simulink model "Quat_Test_v3"  (Simulink 7.5)
settings: Solver=FixedStepDiscrete  StartTime=0.0  StopTime=t(end)  FixedStep=SampleT  RelTol=1e-3
values from neighbouring files (symbols this model uses):
  apSampleTime = 0.01    [demoz2SlugsV5.m]
  QUAT_0 = DCM2Quat( R0 )    [demoz2SlugsV5.m]
  SampleT = 0.02    [demoz2SlugsV5.m]
undefined symbols (not defined in the file or in its folder): DiscIntNeverNeededParam
libraries: simulink x11, dspmtrx3 x1
settings Model: Creator=Robert  LastModifiedBy=Robert
settings DataIOCC: LimitDataPoints=off

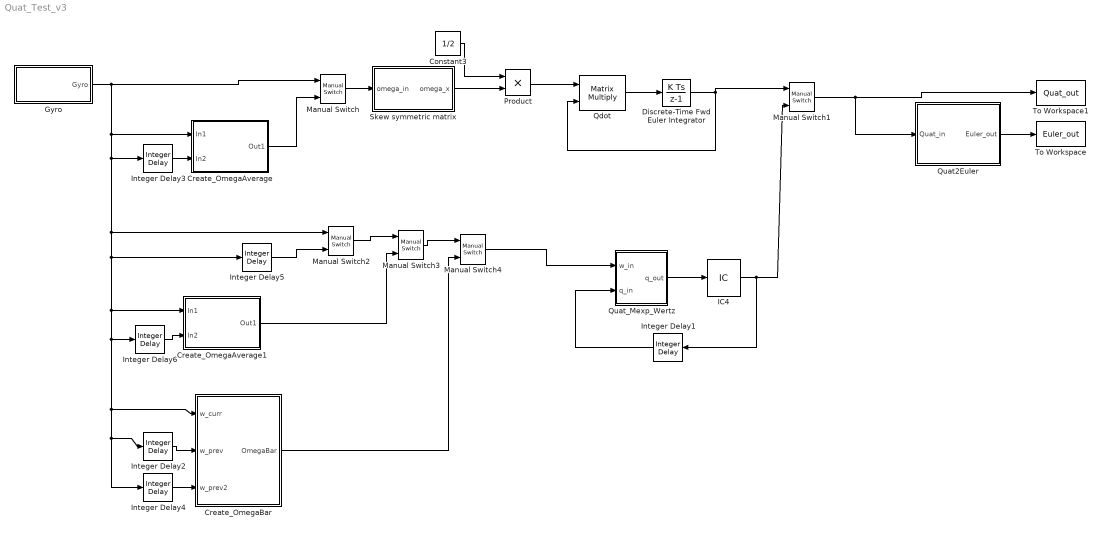
== system Quat_Test_v3 ==
  Constant3 : Constant  Value=1/2  OutDataTypeMode=single  OutDataType=fixdt(1, 16)  OutScaling=2^0  OutDataTypeStr=single
  Create_OmegaAverage : Subsystem
  Create_OmegaAverage1 : Subsystem
  Create_OmegaBar : Subsystem
  Discrete-Time Fwd Euler Integrator : DiscreteIntegrator  InitialCondition=QUAT_0  SampleTime=SampleT  OutDataTypeMode=single  OutDataType=fixdt(1, 16)  OutScaling=2^0  OutDataTypeStr=single  ICPrevOutput=DiscIntNeverNeededParam  ICPrevScaledInput=DiscIntNeverNeededParam
  Gyro : Subsystem
  IC4 : InitialCondition  Value=QUAT_0  SampleTime=apSampleTime
  Integer Delay{1..3,5..6} (5 alike) : simulink/Discrete/Integer Delay  vinit=0.0  samptime=-1  NumDelays=1
  Integer Delay4 : simulink/Discrete/Integer Delay  vinit=0.0  samptime=-1  NumDelays=2
  Manual Switch{,1,3..4} (4 alike) : simulink/Signal Routing/Manual Switch  SystemSampleTime=-1  sw=0  action=0  varsize=off
  Manual Switch2 : simulink/Signal Routing/Manual Switch  SystemSampleTime=-1  sw=1  action=0  varsize=off
  Product : Product  OutDataType=fixdt(1, 16)  OutScaling=2^0  RndMeth=Zero
  Qdot : Product  Multiplication=Matrix(*)  OutDataTypeMode=single  OutDataType=sfix(16)  OutScaling=2^0  OutDataTypeStr=single  SampleTime=SampleT
  Quat2Euler : Subsystem
  Quat_Mexp_Wertz : Subsystem
  Skew symmetric matrix : Subsystem
  To Workspace : ToWorkspace  VariableName=Euler_out  SampleTime=SampleT  SaveFormat=Structure
  To Workspace1 : ToWorkspace  VariableName=Quat_out  SampleTime=SampleT  SaveFormat=Structure
  wires:
  Discrete-Time Fwd Euler Integrator/1 -> Qdot/2, Manual Switch1/1
  Quat2Euler/1(Euler_out) -> To Workspace/1
  Qdot/1 -> Discrete-Time Fwd Euler Integrator/1
  Skew symmetric matrix/1(omega_x) -> Product/2
  Constant3/1 -> Product/1
  Product/1 -> Qdot/1
  Manual Switch/1 -> Skew symmetric matrix/1(omega_in)
  Gyro/1(Gyro) -> Manual Switch/1, Create_OmegaAverage/1(In1), Integer Delay3/1, Manual Switch2/1, Integer Delay5/1, Create_OmegaAverage1/1(In1), Integer Delay6/1, Create_OmegaBar/1(w_curr), Integer Delay2/1, Integer Delay4/1
  Integer Delay3/1 -> Create_OmegaAverage/2(In2)
  Create_OmegaAverage/1(Out1) -> Manual Switch/2
  Integer Delay5/1 -> Manual Switch2/2
  Manual Switch2/1 -> Manual Switch3/1
  Manual Switch3/1 -> Manual Switch4/1
  Integer Delay6/1 -> Create_OmegaAverage1/2(In2)
  Quat_Mexp_Wertz/1(q_out) -> IC4/1
  Manual Switch1/1 -> To Workspace1/1, Quat2Euler/1(Quat_in)
  IC4/1 -> Manual Switch1/2, Integer Delay1/1
  Integer Delay1/1 -> Quat_Mexp_Wertz/2(q_in)
  Manual Switch4/1 -> Quat_Mexp_Wertz/1(w_in)
  Create_OmegaAverage1/1(Out1) -> Manual Switch3/2
  Create_OmegaBar/1(OmegaBar) -> Manual Switch4/2
  Integer Delay2/1 -> Create_OmegaBar/2(w_prev)
  Integer Delay4/1 -> Create_OmegaBar/3(w_prev2)

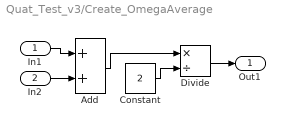
== system Quat_Test_v3/Create_OmegaAverage ==
  In1 : Inport
  In2 : Inport  Port=2
  Add : Sum  OutDataType=fixdt(1, 16)  OutScaling=2^-10
  Constant : Constant  Value=2  OutDataTypeMode=single  OutDataType=fixdt(1, 16)  OutScaling=2^0  OutDataTypeStr=single
  Divide : Product  Inputs=*/  OutDataType=fixdt(1, 16)  OutScaling=2^-10
  Out1 : Outport
  wires:
  Constant/1 -> Divide/2
  Add/1 -> Divide/1
  In1/1 -> Add/1
  In2/1 -> Add/2
  Divide/1 -> Out1/1

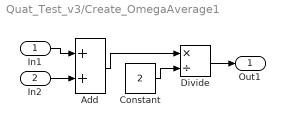
== system Quat_Test_v3/Create_OmegaAverage1 ==
  In1 : Inport
  In2 : Inport  Port=2
  Add : Sum  OutDataType=fixdt(1, 16)  OutScaling=2^-10
  Constant : Constant  Value=2  OutDataTypeMode=single  OutDataType=fixdt(1, 16)  OutScaling=2^0  OutDataTypeStr=single
  Divide : Product  Inputs=*/  OutDataType=fixdt(1, 16)  OutScaling=2^-10
  Out1 : Outport
  wires:
  Divide/1 -> Out1/1
  In2/1 -> Add/2
  In1/1 -> Add/1
  Add/1 -> Divide/1
  Constant/1 -> Divide/2

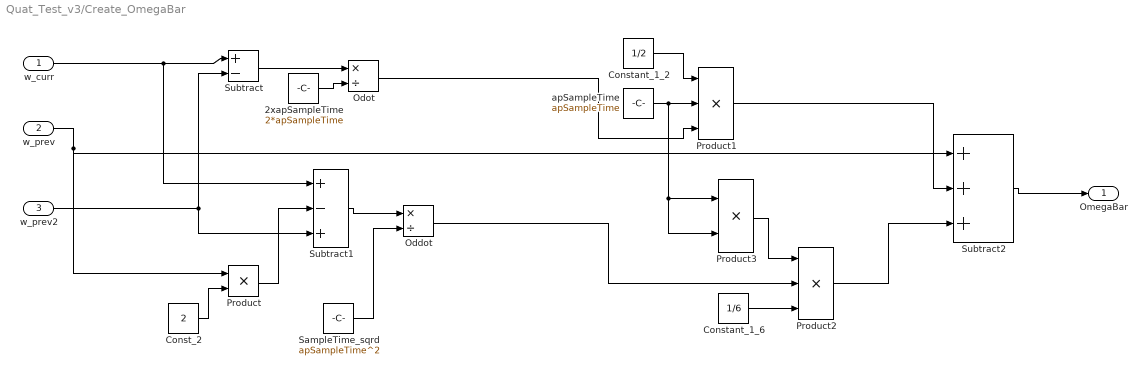
== system Quat_Test_v3/Create_OmegaBar ==
  w_curr : Inport
  w_prev : Inport  Port=2
  w_prev2 : Inport  Port=3
  2xapSampleTime : Constant  Value=2*apSampleTime  OutDataTypeMode=single  OutDataType=fixdt(1, 16)  OutScaling=2^0  OutDataTypeStr=single
  Const_2 : Constant  Value=2  OutDataTypeMode=single  OutDataType=fixdt(1, 16)  OutScaling=2^0  OutDataTypeStr=single
  Constant_1_2 : Constant  Value=1/2  OutDataTypeMode=single  OutDataType=fixdt(1, 16)  OutScaling=2^0  OutDataTypeStr=single
  Constant_1_6 : Constant  Value=1/6  OutDataTypeMode=single  OutDataType=fixdt(1, 16)  OutScaling=2^0  OutDataTypeStr=single
  Oddot : Product  Inputs=*/  OutDataType=fixdt(1, 16)  OutScaling=2^-10
  Odot : Product  Inputs=*/  OutDataType=fixdt(1, 16)  OutScaling=2^-10
  Product : Product  OutDataType=fixdt(1, 16)  OutScaling=2^0  RndMeth=Zero
  Product1 : Product  Inputs=3  OutDataType=fixdt(1, 16)  OutScaling=2^0  RndMeth=Zero
  Product2 : Product  Inputs=3  OutDataType=fixdt(1, 16)  OutScaling=2^0  RndMeth=Zero
  Product3 : Product  OutDataTypeMode=single  OutDataType=fixdt(1, 16)  OutScaling=2^0  OutDataTypeStr=single  SampleTime=apSampleTime  RndMeth=Zero
  SampleTime_sqrd : Constant  Value=apSampleTime^2  OutDataTypeMode=single  OutDataType=fixdt(1, 16)  OutScaling=2^0  OutDataTypeStr=single
  Subtract : Sum  Inputs=+-  OutDataType=fixdt(1, 16)  OutScaling=2^-10
  Subtract1 : Sum  Inputs=+-+  OutDataType=fixdt(1, 16)  OutScaling=2^-10
  Subtract2 : Sum  Inputs=+++  OutDataTypeMode=single  OutDataType=fixdt(1, 16)  OutScaling=2^-10  OutDataTypeStr=single
  apSampleTime : Constant  Value=apSampleTime  OutDataTypeMode=single  OutDataType=fixdt(1, 16)  OutScaling=2^0  OutDataTypeStr=single
  OmegaBar : Outport
  wires:
  w_prev/1 -> Product/1, Subtract2/1
  w_curr/1 -> Subtract/1, Subtract1/1
  w_prev2/1 -> Subtract/2, Subtract1/3
  Subtract/1 -> Odot/1
  2xapSampleTime/1 -> Odot/2
  SampleTime_sqrd/1 -> Oddot/2
  Subtract1/1 -> Oddot/1
  Const_2/1 -> Product/2
  Product/1 -> Subtract1/2
  Subtract2/1 -> OmegaBar/1
  Constant_1_2/1 -> Product1/1
  apSampleTime/1 -> Product1/2, Product3/1, Product3/2
  Odot/1 -> Product1/3
  Product1/1 -> Subtract2/2
  Constant_1_6/1 -> Product2/3
  Product3/1 -> Product2/1
  Oddot/1 -> Product2/2
  Product2/1 -> Subtract2/3

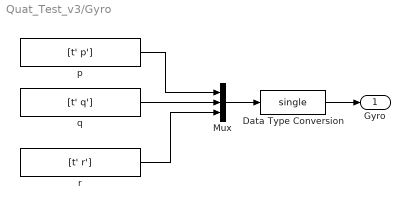
== system Quat_Test_v3/Gyro ==
  Data Type Conversion : DataTypeConversion  OutDataTypeMode=single  OutDataType=sfix(16)  OutScaling=2^0  OutDataTypeStr=single  SampleTime=SampleT
  Mux : Mux  Inputs=3
  p : FromWorkspace  VariableName=[t' p']  SampleTime=SampleT  Interpolate=off  OutputAfterFinalValue=Setting to zero
  q : FromWorkspace  VariableName=[t' q']  SampleTime=0.01  OutputAfterFinalValue=Setting to zero
  r : FromWorkspace  VariableName=[t' r']  SampleTime=0.01  OutputAfterFinalValue=Setting to zero
  Gyro : Outport  OutDataType=sfix(16)  OutScaling=2^0
  wires:
  Data Type Conversion/1 -> Gyro/1
  Mux/1 -> Data Type Conversion/1
  r/1 -> Mux/3
  q/1 -> Mux/2
  p/1 -> Mux/1

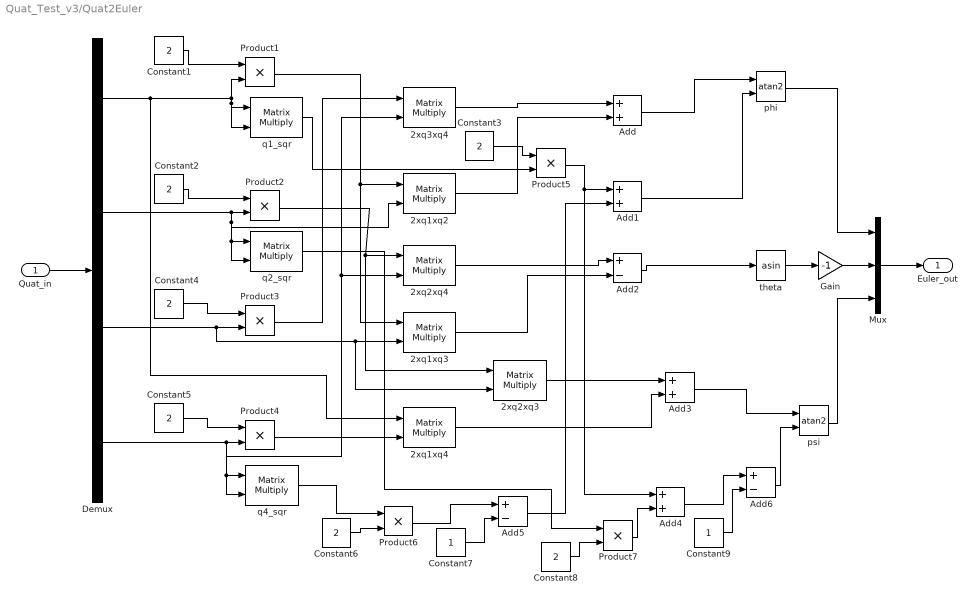
== system Quat_Test_v3/Quat2Euler ==
  Quat_in : Inport  OutDataType=fixdt(1, 16)  OutScaling=2^0
  2xq1xq2 : Product  Multiplication=Matrix(*)  OutDataTypeMode=single  OutDataType=sfix(16)  OutScaling=2^0  OutDataTypeStr=single  SampleTime=SampleT
  2xq1xq3 : Product  Multiplication=Matrix(*)  OutDataTypeMode=single  OutDataType=sfix(16)  OutScaling=2^0  OutDataTypeStr=single  SampleTime=SampleT
  2xq1xq4 : Product  Multiplication=Matrix(*)  OutDataTypeMode=single  OutDataType=sfix(16)  OutScaling=2^0  OutDataTypeStr=single  SampleTime=SampleT
  2xq2xq3 : Product  Multiplication=Matrix(*)  OutDataTypeMode=single  OutDataType=sfix(16)  OutScaling=2^0  OutDataTypeStr=single  SampleTime=SampleT
  2xq2xq4 : Product  Multiplication=Matrix(*)  OutDataTypeMode=single  OutDataType=sfix(16)  OutScaling=2^0  OutDataTypeStr=single  SampleTime=SampleT
  2xq3xq4 : Product  Multiplication=Matrix(*)  OutDataTypeMode=single  OutDataType=sfix(16)  OutScaling=2^0  OutDataTypeStr=single  SampleTime=SampleT
  Add{,1,3..4} (4 alike) : Sum  AccumDataTypeStr=single  OutDataType=fixdt(1, 16)  OutScaling=2^-10  SampleTime=SampleT
  Add2 : Sum  Inputs=+-  AccumDataTypeStr=single  OutDataType=fixdt(1, 16)  OutScaling=2^-10  SampleTime=SampleT
  Add5 : Sum  Inputs=+-  AccumDataTypeStr=single  OutDataType=fixdt(1, 16)  OutScaling=2^-10
  Add6 : Sum  Inputs=+-  AccumDataTypeStr=single  OutDataType=fixdt(1, 16)  OutScaling=2^-10
  Constant{1..6,8} (7 alike) : Constant  Value=2  OutDataTypeMode=single  OutDataType=fixdt(1, 16)  OutScaling=2^0  OutDataTypeStr=single
  Constant7 : Constant  OutDataTypeMode=single  OutDataType=fixdt(1, 16)  OutScaling=2^0  OutDataTypeStr=single
  Constant9 : Constant  OutDataTypeMode=single  OutDataType=fixdt(1, 16)  OutScaling=2^0  OutDataTypeStr=single
  Demux : Demux
  Gain : Gain  Gain=-1  ParameterDataType=fixdt(1, 16)  ParameterScaling=2^0  OutDataType=fixdt(1, 16)  OutScaling=2^0
  Mux : Mux  Inputs=3
  Product{1..7} (7 alike) : Product  OutDataType=fixdt(1, 16)  OutScaling=2^0  RndMeth=Zero
  phi : Trigonometry  Operator=atan2
  psi : Trigonometry  Operator=atan2
  q1_sqr : Product  Multiplication=Matrix(*)  OutDataTypeMode=single  OutDataType=sfix(16)  OutScaling=2^0  OutDataTypeStr=single  SampleTime=SampleT
  q2_sqr : Product  Multiplication=Matrix(*)  OutDataTypeMode=single  OutDataType=sfix(16)  OutScaling=2^0  OutDataTypeStr=single  SampleTime=SampleT
  q4_sqr : Product  Multiplication=Matrix(*)  OutDataTypeMode=single  OutDataType=sfix(16)  OutScaling=2^0  OutDataTypeStr=single  SampleTime=SampleT
  theta : Trigonometry  Operator=asin
  Euler_out : Outport  OutDataType=fixdt(1, 16)  OutScaling=2^0
  wires:
  psi/1 -> Mux/3
  Gain/1 -> Mux/2
  phi/1 -> Mux/1
  theta/1 -> Gain/1
  Quat_in/1 -> Demux/1
  Mux/1 -> Euler_out/1
  Constant5/1 -> Product4/1
  Constant4/1 -> Product3/1
  Constant2/1 -> Product2/1
  Constant1/1 -> Product1/1
  Demux/1 -> Product1/2, q1_sqr/1, q1_sqr/2, 2xq1xq4/1
  Demux/2 -> Product2/2, q2_sqr/1, q2_sqr/2, 2xq1xq2/2
  Demux/3 -> Product3/2, 2xq1xq3/2, 2xq2xq3/2
  Demux/4 -> Product4/2, q4_sqr/1, q4_sqr/2, 2xq3xq4/2, 2xq2xq4/2
  Product3/1 -> 2xq3xq4/1
  2xq3xq4/1 -> Add/1
  Add/1 -> phi/1
  Product1/1 -> 2xq1xq2/1, 2xq1xq3/1
  2xq1xq2/1 -> Add/2
  q1_sqr/1 -> Product5/2
  Constant3/1 -> Product5/1
  Product5/1 -> Add1/1, Add4/1
  q4_sqr/1 -> Product6/1
  Constant6/1 -> Product6/2
  Constant7/1 -> Add5/2
  Product6/1 -> Add5/1
  Add5/1 -> Add1/2
  Add1/1 -> phi/2
  Product2/1 -> 2xq2xq4/1, 2xq2xq3/1
  2xq2xq4/1 -> Add2/1
  2xq1xq3/1 -> Add2/2
  Add2/1 -> theta/1
  Add3/1 -> psi/1
  2xq2xq3/1 -> Add3/1
  Product4/1 -> 2xq1xq4/2
  2xq1xq4/1 -> Add3/2
  Constant8/1 -> Product7/2
  Product7/1 -> Add4/2
  q2_sqr/1 -> Product7/1
  Constant9/1 -> Add6/2
  Add4/1 -> Add6/1
  Add6/1 -> psi/2

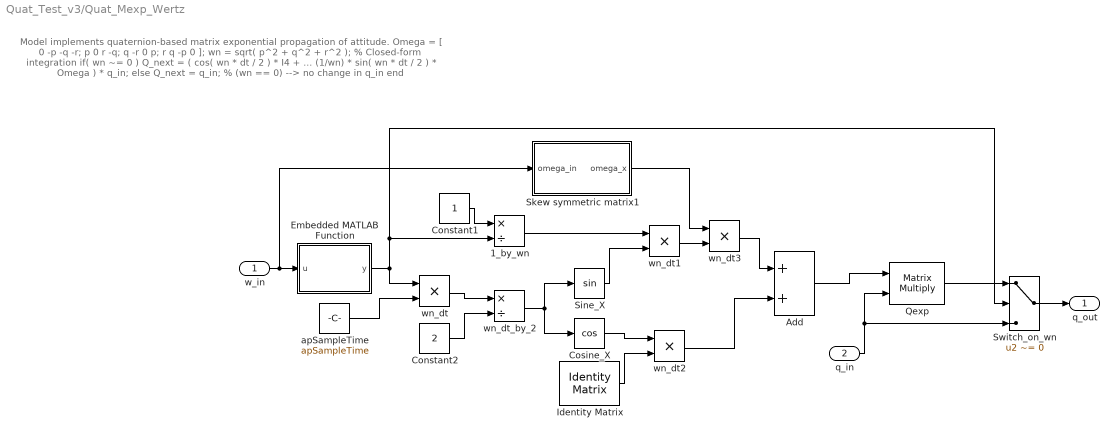
== system Quat_Test_v3/Quat_Mexp_Wertz ==
  note: Model implements quaternion-based matrix exponential propagation of attitude.
      | Omega = [ 0 -p -q -r; p 0 r -q; q -r 0 p; r q -p 0 ];
      | wn = sqrt( p^2 + q^2 + r^2 );
      |
      | % Closed-form integration
      | if( wn ~= 0 )
      |     Q_next = (   cos( wn * dt / 2 ) * I4 + ...
      |         (1/wn) * sin( wn * dt / 2 ) * Omega ) * q_in;
      | else
      |     Q_next = q_in; % (wn == 0) --> no change in q_in
      | end
  w_in : Inport  OutDataType=fixdt(1, 16)  OutScaling=2^0
  q_in : Inport  Port=2  OutDataType=fixdt(1, 16)  OutScaling=2^0
  1_by_wn : Product  Inputs=*/  OutDataType=fixdt(1, 16)  OutScaling=2^-10
  Add : Sum  OutDataTypeMode=single  OutDataType=fixdt(1, 16)  OutScaling=2^-10  OutDataTypeStr=single  SampleTime=apSampleTime
  Constant1 : Constant  OutDataTypeMode=single  OutDataType=fixdt(1, 16)  OutScaling=2^0  OutDataTypeStr=single
  Constant2 : Constant  Value=2  OutDataTypeMode=single  OutDataType=fixdt(1, 16)  OutScaling=2^0  OutDataTypeStr=single
  Cosine_X : Trigonometry  Operator=cos
  Embedded MATLAB Function : Stateflow chart  TreatAsAtomicUnit=on
  Identity Matrix : dspmtrx3/Identity Matrix  Inherit=off  N=4  Ts=apSampleTime  dataType=single  isSigned=on  wordLen=16  udDataType=sfix(16)  fracBitsMode=Best precision  numFracBits=15
  Qexp : Product  Multiplication=Matrix(*)  OutDataTypeMode=single  OutDataType=sfix(16)  OutScaling=2^0  OutDataTypeStr=single  SampleTime=SampleT
  Sine_X : Trigonometry
  Skew symmetric matrix1 : Subsystem
  Switch_on_wn : Switch  Criteria=u2 ~= 0  OutDataTypeMode=single  OutDataType=fixdt(1, 16)  OutScaling=2^0  OutDataTypeStr=single
  apSampleTime : Constant  Value=apSampleTime  OutDataTypeMode=single  OutDataType=fixdt(1, 16)  OutScaling=2^0  OutDataTypeStr=single
  wn_dt{,1..3} (4 alike) : Product  OutDataType=fixdt(1, 16)  OutScaling=2^0  RndMeth=Zero
  wn_dt_by_2 : Product  Inputs=*/  OutDataType=fixdt(1, 16)  OutScaling=2^-10
  q_out : Outport  OutDataType=fixdt(1, 16)  OutScaling=2^0
  wires:
  Embedded MATLAB Function/1(y) -> wn_dt/1, 1_by_wn/2, Switch_on_wn/2
  apSampleTime/1 -> wn_dt/2
  w_in/1 -> Embedded MATLAB Function/1(u), Skew symmetric matrix1/1(omega_in)
  wn_dt/1 -> wn_dt_by_2/1
  Constant2/1 -> wn_dt_by_2/2
  wn_dt_by_2/1 -> Sine_X/1, Cosine_X/1
  Constant1/1 -> 1_by_wn/1
  Sine_X/1 -> wn_dt1/2
  1_by_wn/1 -> wn_dt1/1
  wn_dt1/1 -> wn_dt3/2
  wn_dt3/1 -> Add/1
  Cosine_X/1 -> wn_dt2/1
  Identity Matrix/1 -> wn_dt2/2
  wn_dt2/1 -> Add/2
  Skew symmetric matrix1/1(omega_x) -> wn_dt3/1
  Qexp/1 -> Switch_on_wn/1
  Add/1 -> Qexp/1
  q_in/1 -> Qexp/2, Switch_on_wn/3
  Switch_on_wn/1 -> q_out/1

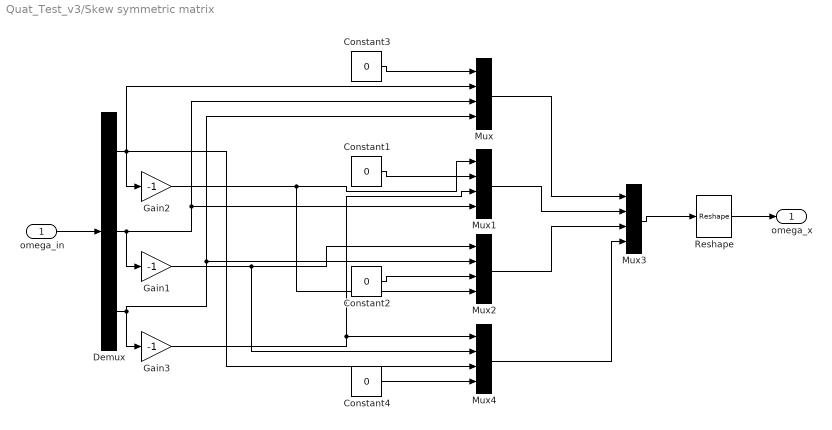
== system Quat_Test_v3/Skew symmetric matrix ==
  omega_in : Inport  DataType=single  OutDataType=fixdt(1, 16)  OutScaling=2^0  OutDataTypeStr=single
  Constant{1..4} (4 alike) : Constant  Value=0  OutDataTypeMode=single  OutDataType=fixdt(1, 16)  OutScaling=2^0  OutDataTypeStr=single
  Demux : Demux  Outputs=3
  Gain1 : Gain  Gain=-1  ParameterDataType=fixdt(1, 16)  ParameterScaling=2^0  OutDataTypeMode=single  OutDataType=fixdt(1, 16)  OutScaling=2^0  OutDataTypeStr=single
  Gain2 : Gain  Gain=-1  ParameterDataType=fixdt(1, 16)  ParameterScaling=2^0  OutDataTypeMode=single  OutDataType=fixdt(1, 16)  OutScaling=2^0  OutDataTypeStr=single
  Gain3 : Gain  Gain=-1  ParameterDataType=fixdt(1, 16)  ParameterScaling=2^0  OutDataTypeMode=single  OutDataType=fixdt(1, 16)  OutScaling=2^0  OutDataTypeStr=single
  Mux{,1..4} (5 alike) : Mux
  Reshape : Reshape  OutputDimensionality=Customize  OutputDimensions=[4,4]
  omega_x : Outport  DataType=single  OutDataType=fixdt(1, 16)  OutScaling=2^0  OutDataTypeStr=single
  wires:
  Gain1/1 -> Mux4/2, Mux2/1
  Gain3/1 -> Mux4/1, Mux1/3
  Gain2/1 -> Mux2/4, Mux1/1
  Mux3/1 -> Reshape/1
  Reshape/1 -> omega_x/1
  omega_in/1 -> Demux/1
  Mux/1 -> Mux3/1
  Mux1/1 -> Mux3/2
  Mux2/1 -> Mux3/3
  Mux4/1 -> Mux3/4
  Constant4/1 -> Mux4/4
  Constant2/1 -> Mux2/3
  Constant1/1 -> Mux1/2
  Constant3/1 -> Mux/1
  Demux/1 -> Mux4/3, Mux/2, Gain2/1
  Demux/2 -> Mux1/4, Mux/3, Gain1/1
  Demux/3 -> Mux2/2, Mux/4, Gain3/1

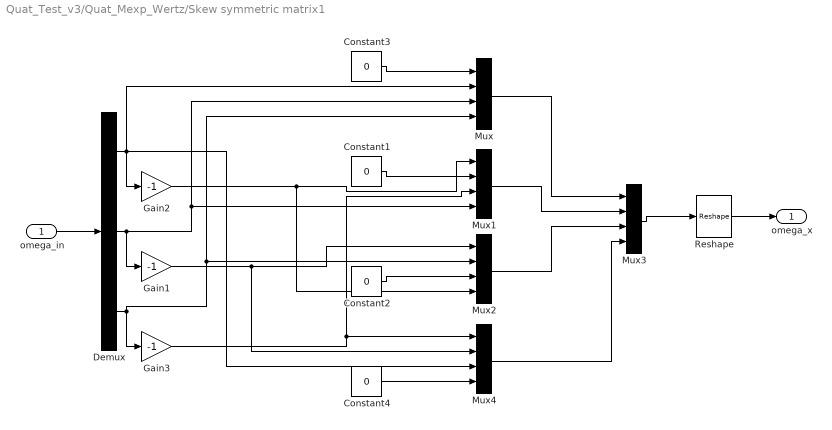
== system Quat_Test_v3/Quat_Mexp_Wertz/Skew symmetric matrix1 ==
  omega_in : Inport  DataType=single  OutDataType=fixdt(1, 16)  OutScaling=2^0  OutDataTypeStr=single
  Constant{1..4} (4 alike) : Constant  Value=0  OutDataTypeMode=single  OutDataType=fixdt(1, 16)  OutScaling=2^0  OutDataTypeStr=single
  Demux : Demux  Outputs=3
  Gain1 : Gain  Gain=-1  ParameterDataType=fixdt(1, 16)  ParameterScaling=2^0  OutDataTypeMode=single  OutDataType=fixdt(1, 16)  OutScaling=2^0  OutDataTypeStr=single
  Gain2 : Gain  Gain=-1  ParameterDataType=fixdt(1, 16)  ParameterScaling=2^0  OutDataTypeMode=single  OutDataType=fixdt(1, 16)  OutScaling=2^0  OutDataTypeStr=single
  Gain3 : Gain  Gain=-1  ParameterDataType=fixdt(1, 16)  ParameterScaling=2^0  OutDataTypeMode=single  OutDataType=fixdt(1, 16)  OutScaling=2^0  OutDataTypeStr=single
  Mux{,1..4} (5 alike) : Mux
  Reshape : Reshape  OutputDimensionality=Customize  OutputDimensions=[4,4]
  omega_x : Outport  DataType=single  OutDataType=fixdt(1, 16)  OutScaling=2^0  OutDataTypeStr=single
  wires:
  Demux/3 -> Gain3/1, Mux/4, Mux2/2
  Demux/2 -> Gain1/1, Mux/3, Mux1/4
  Demux/1 -> Gain2/1, Mux/2, Mux4/3
  Constant3/1 -> Mux/1
  Constant1/1 -> Mux1/2
  Constant2/1 -> Mux2/3
  Constant4/1 -> Mux4/4
  Mux4/1 -> Mux3/4
  Mux2/1 -> Mux3/3
  Mux1/1 -> Mux3/2
  Mux/1 -> Mux3/1
  omega_in/1 -> Demux/1
  Reshape/1 -> omega_x/1
  Mux3/1 -> Reshape/1
  Gain2/1 -> Mux1/1, Mux2/4
  Gain3/1 -> Mux1/3, Mux4/1
  Gain1/1 -> Mux2/1, Mux4/2

== matlab function Quat_Mexp_Wertz/Embedded MATLAB Function ==
  data: u input double; y output double
function y = GetNorm(u)
%#eml
% Function returns the 2-norm of the input argument.

y = norm(u);
